simulink model "Control_System_2"  (R2021a)
settings: Solver=VariableStepAuto  StartTime=0.0  StopTime=10.0  RelTol=1e-3
settings Model: Creator=my computer  LastModifiedBy=my computer

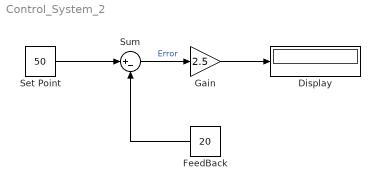
== system Control_System_2 ==
  Display : Display
  FeedBack : Constant  Value=20
  Gain : Gain  Gain=2.5
  Set Point : Constant  Value=50
  Sum : Sum  Inputs=|+-
  wires:
  FeedBack/1 -> Sum/2
  Set Point/1 -> Sum/1
  Sum/1 -> Gain/1  "Error"
  Gain/1 -> Display/1
